simulink model "MobileManipulatorMaster"  (R2016a)
settings: Solver=FixedStepDiscrete  StartTime=0.0  StopTime=inf  FixedStep=.001  RelTol=1e-3
libraries: LibrarySimulinkSAS x1, aerolibanimutils x1, dspnetwork x1
settings Model: Creator=santd  LastModifiedBy=santd

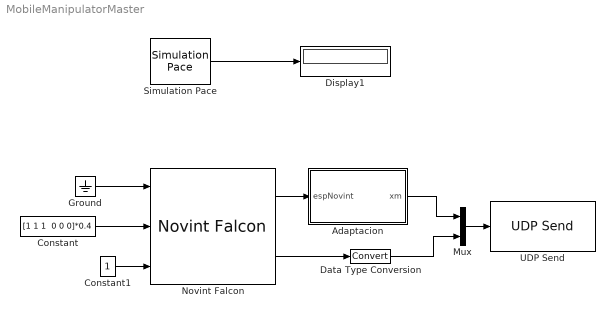
== system MobileManipulatorMaster ==
  Adaptacion : Subsystem
  Constant : Constant  Value="[1 1 1  0 0 0]*0.4"
  Constant1 : Constant  OutDataTypeStr=boolean
  Data Type Conversion : DataTypeConversion
  Display1 : Display
  Ground : Ground
  Mux : Mux  Inputs=2
  Novint Falcon : LibrarySimulinkSAS/Novint Falcon  dev=1
  Simulation Pace : aerolibanimutils/Simulation Pace  SimulationPace=1  SleepMode=MATLAB Thread  OutputPaceError=on  SampleTime=-1
  UDP Send : dspnetwork/UDP Send  remoteURL='255.255.255.255'  remotePort=24100  localURL='0.0.0.0'  localPortSource=Automatically determine  localPort=-1  sampletime=-1  blockPlatform=[]  separateLengthPort=0
  wires:
  Novint Falcon/1 -> Adaptacion/1(espNovint)
  Constant/1 -> Novint Falcon/2
  Constant1/1 -> Novint Falcon/3
  Simulation Pace/1 -> Display1/1
  Adaptacion/1(xm) -> Mux/1
  Novint Falcon/2 -> Data Type Conversion/1
  Mux/1 -> UDP Send/1
  Data Type Conversion/1 -> Mux/2
  Ground/1 -> Novint Falcon/1

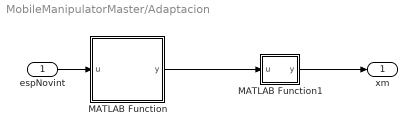
== system MobileManipulatorMaster/Adaptacion ==
  espNovint : Inport
  MATLAB Function : MATLAB Function  TreatAsAtomicUnit=on
  MATLAB Function1 : MATLAB Function  TreatAsAtomicUnit=on
  xm : Outport
  wires:
  espNovint/1 -> MATLAB Function/1(u)
  MATLAB Function/1(y) -> MATLAB Function1/1(u)
  MATLAB Function1/1(y) -> xm/1

== matlab function MobileManipulatorMaster/Adaptacion/MATLAB Function1 ==
  data: u input; y output
function y = fcn(u)
%#codegen

y = u(1:3);

== matlab function MobileManipulatorMaster/Adaptacion/MATLAB Function ==
  data: u input; y output
function y = fcn(u)
y=zeros(6,1);
y(1)= -u(3);%-1;  %x
y(2)= u(1);    %y
y(3)=  u(2);    %z
y(4)= -u(4);
y(5)= -u(5);
y(6)=  u(6);
y=y/100;%[cm->m]
